simulink model "Bulk_FL_PP_SE_Sim"  (R2015a)
settings: Solver=ode5  StartTime=0.0  StopTime=tf  FixedStep=t_step  RelTol=1e-3
values from neighbouring files (symbols this model uses):
  A = [ -1/(R*Cp), 1/Cp; -1/L, 0]    [Bulk_FL_PP_SE.m]    (also in Bulk_SM_PP_SE.m; Bulk_SM_SM_SE.m)
  B = [0;  Vi/L]    [Bulk_FL_PP_SE.m]    (also in Bulk_SM_PP_SE.m; Bulk_SM_SM_SE.m)
  C = [1, 0]    [Bulk_FL_PP_SE.m]    (also in Bulk_SM_PP_SE.m; Bulk_SM_SM_SE.m)
  Cp = 50e-6    (= 5e-05)    [BulkMod_SMIA_SMIA.m]    (also in Bulk_FL_PP_SE.m; Bulk_SM_PP_SE.m; Bulk_SM_SM_SE.m)
  DBm = DB * Ts / (2*L)    (= 0.04)    [BulkMod_SMIA_SMIA.m]    (also in Bulk_FL_PP_SE.m; Bulk_SM_PP_SE.m; Bulk_SM_SM_SE.m)
  K0 = sp1 * sp2    [Bulk_FL_PP_SE.m]    (also in Bulk_SM_PP_SE.m)
  K1 = - (sp1 + sp2)    [Bulk_FL_PP_SE.m]    (also in Bulk_SM_PP_SE.m)
  L = 100e-6    (= 0.0001)    [BulkMod_SMIA_SMIA.m]    (also in Bulk_FL_PP_SE.m; Bulk_SM_PP_SE.m; Bulk_SM_SM_SE.m)
  L_fpe = place(A', C', P_obs)'    [Bulk_FL_PP_SE.m]    (also in Bulk_SM_PP_SE.m; Bulk_SM_SM_SE.m)
  R = 100    [BulkMod_SMIA_SMIA.m]    (also in Bulk_FL_PP_SE.m; Bulk_SM_PP_SE.m; Bulk_SM_SM_SE.m)
  Ts = 1e-5    (= 1e-05)    [BulkMod_SMIA_SMIA.m]    (also in Bulk_FL_PP_SE.m; Bulk_SM_PP_SE.m; Bulk_SM_SM_SE.m)
  Vi = 30    [BulkMod_SMIA_SMIA.m]    (also in Bulk_FL_PP_SE.m; Bulk_SM_PP_SE.m; Bulk_SM_SM_SE.m)
libraries: simulink x1
settings Model: Creator=Marcelo  LastModifiedBy=Marcelo

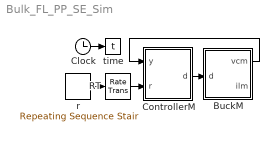
== system Bulk_FL_PP_SE_Sim ==
  BuckM : Subsystem
  Clock : Clock
  ControllerM : Subsystem
  RT : RateTransition  Integrity=off  Deterministic=off  X0=2
  r : simulink/Sources/Repeating Sequence Stair  OutValues=[2, 26, 14].'  tsamp=Tr  OutMin=[]  OutMax=[]  OutDataTypeStr=double  OutputDataTypeScalingMode=double  OutDataType=fixdt(0,8)  ConRadixGroup=Best Precision: Vector-wise  OutScaling=2^-12
  time : ToWorkspace  VariableName=t  SampleTime=-1
  wires:
  Clock/1 -> time/1
  BuckM/1(vcm) -> ControllerM/1(y)
  r/1 -> RT/1
  RT/1 -> ControllerM/2(r)
  ControllerM/1(d) -> BuckM/1(d)

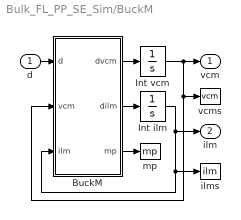
== system Bulk_FL_PP_SE_Sim/BuckM ==
  d : Inport
  BuckM : MATLAB Function  TreatAsAtomicUnit=on
  Int ilm : Integrator  LimitOutput=on  LowerSaturationLimit=0
  Int vcm : Integrator  LimitOutput=on  LowerSaturationLimit=0
  ilms : ToWorkspace  VariableName=ilm  SampleTime=-1
  mp : ToWorkspace  VariableName=mp  SampleTime=-1
  vcms : ToWorkspace  VariableName=vcm  SampleTime=-1
  vcm : Outport
  ilm : Outport  Port=2
  wires:
  BuckM/1(dvcm) -> Int vcm/1
  BuckM/2(dilm) -> Int ilm/1
  Int ilm/1 -> BuckM/3(ilm), ilms/1, ilm/1
  d/1 -> BuckM/1(d)
  Int vcm/1 -> BuckM/2(vcm), vcms/1, vcm/1
  BuckM/3(mp) -> mp/1

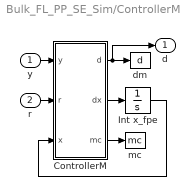
== system Bulk_FL_PP_SE_Sim/ControllerM ==
  y : Inport
  r : Inport  Port=2
  ControllerM : MATLAB Function  TreatAsAtomicUnit=on
  Int x_fpe : Integrator  InitialCondition=[0; 0]  LimitOutput=on  UpperSaturationLimit=[2*Vi; 2*Vi/R]  LowerSaturationLimit=[0; 0]
  dm : ToWorkspace  VariableName=d  SampleTime=-1
  mc : ToWorkspace  VariableName=mc  SampleTime=-1
  d : Outport
  wires:
  ControllerM/1(d) -> d/1, dm/1
  y/1 -> ControllerM/1(y)
  r/1 -> ControllerM/2(r)
  ControllerM/3(mc) -> mc/1
  ControllerM/2(dx) -> Int x_fpe/1
  Int x_fpe/1 -> ControllerM/3(x)

== matlab function Bulk_FL_PP_SE_Sim/BuckM/BuckM ==
  data: d input; dvcm output; vcm input; ilm input; Vi parameter; R parameter; L parameter; Cp parameter; dilm output; Ts parameter; DBm parameter; mp output
function [dvcm, dilm, mp] = fcn(d, vcm, ilm, Vi, R, L, Cp, Ts, DBm)
dvcm = (ilm - vcm/R) / Cp;
ilb = DBm * (Vi - vcm);  % Boundary
if (ilm < ilb) %%%   NONLINEAR   %%%
    dilm = Vi*d/L - 2*ilm*vcm/(d*Ts*(Vi-vcm));
    mp = 0;
else           %%%   LINEAR      %%%
    dilm = (Vi*d - vcm) / L;
    mp = 1;
end

== matlab function Bulk_FL_PP_SE_Sim/ControllerM/ControllerM ==
  data: y input double size=1; d output double size=1; r input double size=1; x input double size=2; dx output double size=2; K1 parameter double size=1; K0 parameter double size=1; R parameter double size=1; Cp parameter double size=1; L parameter; Vi parameter; Ts parameter; DBm parameter; mc output double size=1; A parameter; B parameter; C parameter; L_fpe parameter double size=2
function [d, dx, mc] = fcn(y, r, x, K1, K0, R, Cp, L, Vi, Ts, DBm, A, B, C, L_fpe)
vcm = x(1);
ilm = x(2);
ilb = DBm * (Vi - vcm); % Boundary
if ilm < ilb %%%   NONLINEAR   %%%
    % Controller
    v = - K1 * (ilm - vcm/R) / Cp - K0 * (vcm - r);
    a = L * ((ilm - vcm/R)/(R*Cp) + Cp*v) / (2*Vi);
    b = 2 * ilm * vcm * L / (Vi * Ts * abs(Vi - vcm));
    d = a + sqrt(a^2 + b);
    % Observer
    xs1 = (ilm - vcm/R) / Cp;
    xs2 = Vi*d/L - 2*ilm*vcm/(d*Ts*(Vi-vcm));
    dx = [xs1; xs2] + L_fpe * (y - C*x);
    mc = 0;
else         %%%   LINEAR      %%%
    % Controller
    v = - K1 * (ilm - vcm/R) / Cp - K0 * (vcm - r);
    d = (L * (Cp*v + (ilm - vcm/R) / (R*Cp)) + vcm) / Vi;
    % Observer
    dx = A*x + B*d + L_fpe * (y - C*x);
    mc = 1;
end

if d > 1
    d = 1;
elseif d < 1e-10
    d = 1e-10;
end
